simulink model "BFE_TestHarness"  (Simulink 8.6)
settings: Solver=FixedStepDiscrete  StartTime=0.0  StopTime=3  FixedStep=Ts  RelTol=1e-3
PreLoadFcn:
  | addpath('MBD_Tests')
  | 
  | load('Workspace\EnvVar.mat')
  | run('MBD_Tests\MBD_tests_init.m')
  | if exist('tl_preloadfcn','file'), tl_preloadfcn(gcs,402); end
PostLoadFcn:
  | if exist('tl_postloadfcn','file'), tl_postloadfcn(gcs,402); end
InitFcn:
  | if exist('tlds_init','file'), tlds_init(gcs); end
StartFcn:
  | if exist('tlds_start','file'), tlds_start(gcs); end
StopFcn:
  | if exist('tlds_stop','file'), tlds_stop(gcs); end
undefined symbols (not defined in the file): ddv, Ts, u2, u3, u4
libraries: tllib x11, simulink x8, LIB_TF_G_111 x2, LIB_TF_G_12_StepControl x2, LIB_TF_G_112 x1, LIB_TF_G_113 x1
(part 15 of 17)

== system BFE_TestHarness/BFE_AC_BeltFunctionExecution/Subsystem/BFE_AC_BeltFunctionExecution/BFE_AC_BeltFunctionExecution/BFE_runExecuteStandardSteps/ExecuteStandardSteps/SubsystemConvertOrderToMotorPower/Current_Regulation/Standard Regulation/RescaleMotorMeasure 1lsb = 50mA ==
  MotorCommandSign : Inport  RequirementInfo={} %GIDa_ddc2de95_3bef_4d8e_93b1_f33af8d229ea
  MotorUnsigned : Inport  RequirementInfo={} %GIDa_c6d26590_74e9_40ee_9fc6_c313c8b1f55d  Port=2
  0 Int 16bits : Constant  RequirementInfo={} %GIDa_7831c855_5c9d_4fc0_a40d_65f08d384ac0  Value=ddv('Common/KS16_ZERO')  OutDataTypeStr=uint8  mask(TL_Constant){data={'output',{'variable','Common/KS16_ZERO'},'date',735951.66853826388}}
      settings: CopyFcn=if exist('tl_reset_reviewflag','file')==2,tl_reset_reviewflag(gcbh);end  DeleteFcn=if exist('delete_tlblock','file')==2,delete_tlblock(gcbh);end  NameChangeFcn=if exist('rename_tlblock','file')==2,rename_tlblock(gcbh);end  OpenFcn=if exist('tl_open_blockdlg','file')==2,tl_open_blockdlg(gcbh);else,open_system(gcbh,'parameter');end
      mask Help: eval(['if exist(''tl_online_help'',''file'') == 2, tl_online_help(''Topic'',''TL_Constant''),else, web([''jar:file:///'',matlabroot,''/help/toolbox/simulink/help.jar!/slref/' lower(get_param(gcbh,'Blocktype')) '.html''], ''-helpbrowser''),end'])
      mask Display: plot([-0.05, 1.05, NaN, -0.05, 1.05],[.01, .01, NaN, .99, .99])
  BFE/KU8_PID_mA_RESCALING : Constant  RequirementInfo={} %GIDa_28865132_38f2_4152_8d2a_1d87ea42668e  Value=ddv('BFE/KU8_PID_mA_RESCALING')  OutDataTypeStr=uint8  mask(TL_Constant){data={'output',{'variable','BFE/KU8_PID_mA_RESCALING'},'date',735951.6685378704}}
      settings: CopyFcn=if exist('tl_reset_reviewflag','file')==2,tl_reset_reviewflag(gcbh);end  DeleteFcn=if exist('delete_tlblock','file')==2,delete_tlblock(gcbh);end  NameChangeFcn=if exist('rename_tlblock','file')==2,rename_tlblock(gcbh);end  OpenFcn=if exist('tl_open_blockdlg','file')==2,tl_open_blockdlg(gcbh);else,open_system(gcbh,'parameter');end
      mask Help: eval(['if exist(''tl_online_help'',''file'') == 2, tl_online_help(''Topic'',''TL_Constant''),else, web([''jar:file:///'',matlabroot,''/help/toolbox/simulink/help.jar!/slref/' lower(get_param(gcbh,'Blocktype')) '.html''], ''-helpbrowser''),end'])
      mask Display: plot([-0.05, 1.05, NaN, -0.05, 1.05],[.01, .01, NaN, .99, .99])
  KUC_ONE : Constant  RequirementInfo={} %GIDa_d9d69a7f_538e_4932_bf64_59549179e9a4  Value=ddv('Common/KU8_ONE')  OutDataTypeStr=uint8  mask(TL_Constant){data={'output',{'variable','Common/KU8_ONE'},'date',735951.66853748844}}
      settings: CopyFcn=if exist('tl_reset_reviewflag','file')==2,tl_reset_reviewflag(gcbh);end  DeleteFcn=if exist('delete_tlblock','file')==2,delete_tlblock(gcbh);end  NameChangeFcn=if exist('rename_tlblock','file')==2,rename_tlblock(gcbh);end  OpenFcn=if exist('tl_open_blockdlg','file')==2,tl_open_blockdlg(gcbh);else,open_system(gcbh,'parameter');end
      mask Help: eval(['if exist(''tl_online_help'',''file'') == 2, tl_online_help(''Topic'',''TL_Constant''),else, web([''jar:file:///'',matlabroot,''/help/toolbox/simulink/help.jar!/slref/' lower(get_param(gcbh,'Blocktype')) '.html''], ''-helpbrowser''),end'])
      mask Display: plot([-0.05, 1.05, NaN, -0.05, 1.05],[.01, .01, NaN, .99, .99])
  Product : Product  RequirementInfo={} %GIDa_989e5ae6_3fb7_483c_9c3c_230268316b82  Inputs=*/  OutDataTypeStr=uint32  RndMeth=Zero  mask(TL_Product){data={'output',{'type','UInt16'},'date',735951.66853710648}}
      settings: CopyFcn=if exist('tl_reset_reviewflag','file')==2,tl_reset_reviewflag(gcbh);end  DeleteFcn=if exist('delete_tlblock','file')==2,delete_tlblock(gcbh);end  NameChangeFcn=if exist('rename_tlblock','file')==2,rename_tlblock(gcbh);end  OpenFcn=if exist('tl_open_blockdlg','file')==2,tl_open_blockdlg(gcbh);else,open_system(gcbh,'parameter');end
      mask Help: eval(['if exist(''tl_online_help'',''file'') == 2, tl_online_help(''Topic'',''TL_Product''),else, web([''jar:file:///'',matlabroot,''/help/toolbox/simulink/help.jar!/slref/' lower(get_param(gcbh,'Blocktype')) '.html''], ''-helpbrowser''),end'])
      mask Display: plot([-0.05, 1.05, NaN, -0.05, 1.05],[.01, .01, NaN, .99, .99])
  Product1 : Product  RequirementInfo={} %GIDa_e457ca61_25f4_4aaf_857a_6a7a18ea8d4b  Inputs=**  OutDataTypeStr=int16  RndMeth=Zero  mask(TL_Product){data={'date',735951.66853673616}}
      settings: CopyFcn=if exist('tl_reset_reviewflag','file')==2,tl_reset_reviewflag(gcbh);end  DeleteFcn=if exist('delete_tlblock','file')==2,delete_tlblock(gcbh);end  NameChangeFcn=if exist('rename_tlblock','file')==2,rename_tlblock(gcbh);end  OpenFcn=if exist('tl_open_blockdlg','file')==2,tl_open_blockdlg(gcbh);else,open_system(gcbh,'parameter');end
      mask Help: eval(['if exist(''tl_online_help'',''file'') == 2, tl_online_help(''Topic'',''TL_Product''),else, web([''jar:file:///'',matlabroot,''/help/toolbox/simulink/help.jar!/slref/' lower(get_param(gcbh,'Blocktype')) '.html''], ''-helpbrowser''),end'])
      mask Display: plot([-0.05, 1.05, NaN, -0.05, 1.05],[.01, .01, NaN, .99, .99])
  Relational Operator : RelationalOperator  RequirementInfo={} %GIDa_0667d066_9ed8_4393_bb31_70e18b8dd437  Operator===  OutDataTypeStr=boolean  mask(TL_RelationalOperator){data={'date',735951.66853637737}}
      settings: DeleteFcn=if exist('delete_tlblock','file')==2,delete_tlblock(gcbh);end  NameChangeFcn=if exist('rename_tlblock','file')==2,rename_tlblock(gcbh);end  OpenFcn=if exist('tl_open_blockdlg','file')==2,tl_open_blockdlg(gcbh);else,open_system(gcbh,'parameter');end
      mask Help: eval(['if exist(''tl_online_help'',''file'') == 2, tl_online_help(''Topic'',''TL_RelationalOperator''),else, web([''jar:file:///'',matlabroot,''/help/toolbox/simulink/help.jar!/slref/' lower(get_param(gcbh,'Blocktype')) '.html''], ''-helpbrowser''),end'])
      mask Display: plot([-0.05, 1.05, NaN, -0.05, 1.05],[.01, .01, NaN, .99, .99])
  Sign : Signum  RequirementInfo={} %GIDa_e8c68066_07cd_49ad_8f47_c39297ac8a64  mask(TL_Signum){data={'date',735951.6685361343}}
      settings: DeleteFcn=if exist('delete_tlblock','file')==2,delete_tlblock(gcbh);end  NameChangeFcn=if exist('rename_tlblock','file')==2,rename_tlblock(gcbh);end  OpenFcn=if exist('tl_open_blockdlg','file')==2,tl_open_blockdlg(gcbh);else,open_system(gcbh,'parameter');end
      mask Help: eval(['if exist(''tl_online_help'',''file'') == 2, tl_online_help(''Topic'',''TL_Signum''),else, web([''jar:file:///'',matlabroot,''/help/toolbox/simulink/help.jar!/slref/' lower(get_param(gcbh,'Blocktype')) '.html''], ''-helpbrowser''),end'])
      mask Display: plot([-0.05, 1.05, NaN, -0.05, 1.05],[.01, .01, NaN, .99, .99])
  Switch : Switch  RequirementInfo={} %GIDa_e47adc39_9841_47d4_9acc_035cc38b4113  Criteria=u2 ~= 0  mask(TL_Switch){data={'output',{'type','Int8'},'date',735951.66853584489}}
      settings: CopyFcn=if exist('tl_reset_reviewflag','file')==2,tl_reset_reviewflag(gcbh);end  DeleteFcn=if exist('delete_tlblock','file')==2,delete_tlblock(gcbh);end  NameChangeFcn=if exist('rename_tlblock','file')==2,rename_tlblock(gcbh);end  OpenFcn=if exist('tl_open_blockdlg','file')==2,tl_open_blockdlg(gcbh);else,open_system(gcbh,'parameter');end
      mask Help: eval(['if exist(''tl_online_help'',''file'') == 2, tl_online_help(''Topic'',''TL_Switch''),else, web([''jar:file:///'',matlabroot,''/help/toolbox/simulink/help.jar!/slref/' lower(get_param(gcbh,'Blocktype')) '.html''], ''-helpbrowser''),end'])
      mask Display: plot([-0.05, 1.05, NaN, -0.05, 1.05],[.01, .01, NaN, .99, .99])
  s16MotorCurrent : Outport  RequirementInfo={} %GIDa_bea6628c_dfa8_47c5_b18b_49264848b5ef
  wires:
  MotorCommandSign/1 -> Sign/1, Relational Operator/2
  Sign/1 -> Switch/3
  0 Int 16bits/1 -> Relational Operator/1
  Relational Operator/1 -> Switch/2
  KUC_ONE/1 -> Switch/1
  Product/1 -> Product1/2
  Switch/1 -> Product1/1
  Product1/1 -> s16MotorCurrent/1
  MotorUnsigned/1 -> Product/1
  BFE/KU8_PID_mA_RESCALING/1 -> Product/2

== system BFE_TestHarness/BFE_AC_BeltFunctionExecution/Subsystem/BFE_AC_BeltFunctionExecution/BFE_AC_BeltFunctionExecution/BFE_runExecuteStandardSteps/ExecuteStandardSteps/SubsystemConvertOrderToMotorPower/RescaleOrderType/If Action Subsystem/8Bit Decoder ==
  U8in : Inport  RequirementInfo={} %GIDa_cca83995_da78_4ddb_b2c1_85f13c6d35e0
  8Bit Decoder : S-Function  RequirementInfo={} %GIDa_b6337983_b2e1_41bd_ae7f_dd9ba8b00acd  FunctionName=u8_bit_decoder_flp  Parameters=dt  SFunctionDeploymentMode=off  EnableBusSupport=off  mask(TL_CustomCode){data={'#state',0,'#param',0,'#work',0,'#output',8,'#logdata',8,'codefile','u8_bit_decoder.c','output#1',{'name','$S_$B_bit7','varname','bit7','type','Bool'},'output#2',{'name','$S_$B_bit6','varname','bit6','type','Bool'},'output#3',{'name','$S_$B_bit5','varname','bit5','type','Bool'},'output#4',{'name','$S_$B_bit4','varname','bit4','type','Bool'},'output#5',{'name','$S_$B_bit3','varname','bit3','type','Bool'},'output#6',{'name','$S_$B_bit2','varname','bit2','type','Bool'},'output#7',{'name','$S_$B_bit1','varname','bit1','type','Bool'},'output#8',{'name','$S_$B_bit0','varname','bit0','type','Bool'},'input',{'name','$S_$B_in','varname','u8in','type','UInt8'},'date',735951.66851649305}, dt=-1}
      mask help:
      | TargetLink Custom Code block:
      | Allows to insert custom code into a TargetLink application.
      settings: DeleteFcn=if exist('delete_tlblock','file')==2,delete_tlblock(gcbh);end  NameChangeFcn=if exist('rename_tlblock','file')==2,rename_tlblock(gcbh);end  OpenFcn=if exist('tl_open_blockdlg','file')==2,tl_open_blockdlg(gcbh);else,open_system(gcbh,'mask');end
      mask Help: eval('if exist(''tl_online_help'',''file'') == 2, tl_online_help(''Topic'',get_param(gcbh,''MaskType'')),end')
      mask Display:
      | plot([-0.05, 1.05, NaN, -0.05, 1.05],[.01, .01, NaN, .99, .99])
      | ; disp('u8_bit_decoder.c');port_label('input',1,'u8in');port_label('output',1,'bit7');port_label('output',2,'bit6');port_label('output',3,'bit5');port_label('output',4,'bit4');port_label('output',5,'bit3');port_label('output',6,'bit2');port_label('output',7,'bit1');port_label('output',8,'bit0');
  Bit7 : Outport  RequirementInfo={} %GIDa_79f6aec0_fcce_435d_ab59_8512532b1b11
  Bit6 : Outport  RequirementInfo={} %GIDa_7cd114c3_d211_44fb_b5cc_00bfdef86dbe  Port=2
  Bit5 : Outport  RequirementInfo={} %GIDa_012c8b96_621a_4aef_ba87_93ec05b55b0e  Port=3
  Bit4 : Outport  RequirementInfo={} %GIDa_16ec1885_4505_4833_8f08_779f3b6e4b74  Port=4
  Bit3 : Outport  RequirementInfo={} %GIDa_052869ce_db0b_4020_8a90_97f9c877a41f  Port=5
  Bit2 : Outport  RequirementInfo={} %GIDa_b38fc457_ade6_4ef7_baf3_aff089c2b6cc  Port=6
  Bit1 : Outport  RequirementInfo={} %GIDa_058fcc24_9702_4f94_b51b_68fafb1f5751  Port=7
  Bit0 : Outport  RequirementInfo={} %GIDa_08d7afe0_9577_46ee_bc11_f47871415acc  Port=8
  wires:
  8Bit Decoder/8 -> Bit0/1
  8Bit Decoder/7 -> Bit1/1
  8Bit Decoder/5 -> Bit3/1
  8Bit Decoder/4 -> Bit4/1
  8Bit Decoder/3 -> Bit5/1
  8Bit Decoder/2 -> Bit6/1
  8Bit Decoder/1 -> Bit7/1
  8Bit Decoder/6 -> Bit2/1
  U8in/1 -> 8Bit Decoder/1

== system BFE_TestHarness/BFE_AC_BeltFunctionExecution/Subsystem/BFE_AC_BeltFunctionExecution/BFE_AC_BeltFunctionExecution/BFE_runExecuteStandardSteps/ExecuteStandardSteps/SubsystemConvertOrderToMotorPower/RescaleOrderType/If Action Subsystem1/8Bit Decoder ==
  U8in : Inport  RequirementInfo={} %GIDa_f8d109da_a7cf_43cb_ba2a_57cff145f4b7
  8Bit Decoder : S-Function  RequirementInfo={} %GIDa_8480970b_d4f1_4300_8228_4b45f48dc331  FunctionName=u8_bit_decoder_flp  Parameters=dt  SFunctionDeploymentMode=off  EnableBusSupport=off  mask(TL_CustomCode){data={'#state',0,'#param',0,'#work',0,'#output',8,'#logdata',8,'codefile','u8_bit_decoder.c','output#1',{'name','$S_$B_bit7','varname','bit7','type','Bool'},'output#2',{'name','$S_$B_bit6','varname','bit6','type','Bool'},'output#3',{'name','$S_$B_bit5','varname','bit5','type','Bool'},'output#4',{'name','$S_$B_bit4','varname','bit4','type','Bool'},'output#5',{'name','$S_$B_bit3','varname','bit3','type','Bool'},'output#6',{'name','$S_$B_bit2','varname','bit2','type','Bool'},'output#7',{'name','$S_$B_bit1','varname','bit1','type','Bool'},'output#8',{'name','$S_$B_bit0','varname','bit0','type','Bool'},'input',{'name','$S_$B_in','varname','u8in','type','UInt8'},'date',735951.66851240746}, dt=-1}
      mask help:
      | TargetLink Custom Code block:
      | Allows to insert custom code into a TargetLink application.
      settings: DeleteFcn=if exist('delete_tlblock','file')==2,delete_tlblock(gcbh);end  NameChangeFcn=if exist('rename_tlblock','file')==2,rename_tlblock(gcbh);end  OpenFcn=if exist('tl_open_blockdlg','file')==2,tl_open_blockdlg(gcbh);else,open_system(gcbh,'mask');end
      mask Help: eval('if exist(''tl_online_help'',''file'') == 2, tl_online_help(''Topic'',get_param(gcbh,''MaskType'')),end')
      mask Display:
      | plot([-0.05, 1.05, NaN, -0.05, 1.05],[.01, .01, NaN, .99, .99])
      | ; disp('u8_bit_decoder.c');port_label('input',1,'u8in');port_label('output',1,'bit7');port_label('output',2,'bit6');port_label('output',3,'bit5');port_label('output',4,'bit4');port_label('output',5,'bit3');port_label('output',6,'bit2');port_label('output',7,'bit1');port_label('output',8,'bit0');
  Bit7 : Outport  RequirementInfo={} %GIDa_b6a5be25_b097_4284_bfb7_90bda14f7695
  Bit6 : Outport  RequirementInfo={} %GIDa_aa108eaf_6e73_4eff_ba0d_ce4b2cb6590f  Port=2
  Bit5 : Outport  RequirementInfo={} %GIDa_69d1ebf5_32de_4abe_9da7_6501e9c80693  Port=3
  Bit4 : Outport  RequirementInfo={} %GIDa_cff7f33f_15aa_4d45_9738_92334b2ad4cb  Port=4
  Bit3 : Outport  RequirementInfo={} %GIDa_10fb33c9_2c3b_4c51_9363_d2d49a1a57a5  Port=5
  Bit2 : Outport  RequirementInfo={} %GIDa_bbd0ff01_8027_4926_b455_dd681fe3b481  Port=6
  Bit1 : Outport  RequirementInfo={} %GIDa_bd4306cc_34c7_4243_b7f7_c39257ab2e00  Port=7
  Bit0 : Outport  RequirementInfo={} %GIDa_bf46a027_ea73_4fa1_ae0f_8a8120def989  Port=8
  wires:
  8Bit Decoder/8 -> Bit0/1
  8Bit Decoder/7 -> Bit1/1
  8Bit Decoder/5 -> Bit3/1
  8Bit Decoder/4 -> Bit4/1
  8Bit Decoder/3 -> Bit5/1
  8Bit Decoder/2 -> Bit6/1
  8Bit Decoder/1 -> Bit7/1
  8Bit Decoder/6 -> Bit2/1
  U8in/1 -> 8Bit Decoder/1

== system BFE_TestHarness/BFE_AC_BeltFunctionExecution/Subsystem/BFE_AC_BeltFunctionExecution/BFE_AC_BeltFunctionExecution/BFE_runExecuteStandardSteps/ExecuteStandardSteps/SubsystemConvertOrderToMotorPower/Current_Regulation/PID Regulation/PID feature enabled/DecidePID_Type ==
  bIsPIDSupplyAllowed : Inport  RequirementInfo={} %GIDa_b8e1bc41_3020_4f94_a10f_5d652f887f66
  bIsPIDMotorAllowed : Inport  RequirementInfo={} %GIDa_6b607d2d_643a_40f6_8b00_11a4c418d8d6  Port=2
  If : If  RequirementInfo={} %GIDa_f4e9c3ed_7e78_4540_80fe_45674d068906  NumInputs=2  IfExpression=u1  ElseIfExpressions=u2
  LastPIDType : Subsystem  RequirementInfo={} %GIDa_54517798_8ca0_4716_b2d4_af0f6596f023  TreatAsAtomicUnit=on
  Logical Operator : Logic  RequirementInfo={} %GIDa_3b220856_3c71_4e5e_b150_6d850348e8ad  AllPortsSameDT=off  OutDataTypeStr=boolean  mask(TL_LogicalOperator){data={'date',735951.66839079862}}
      settings: DeleteFcn=if exist('delete_tlblock','file')==2,delete_tlblock(gcbh);end  NameChangeFcn=if exist('rename_tlblock','file')==2,rename_tlblock(gcbh);end  OpenFcn=if exist('tl_open_blockdlg','file')==2,tl_open_blockdlg(gcbh);else,open_system(gcbh,'parameter');end
      mask Help: eval(['if exist(''tl_online_help'',''file'') == 2, tl_online_help(''Topic'',''TL_LogicalOperator''),else, web([''jar:file:///'',matlabroot,''/help/toolbox/simulink/help.jar!/slref/' lower(get_param(gcbh,'Blocktype')) '.html''], ''-helpbrowser''),end'])
      mask Display: plot([-0.05, 1.05, NaN, -0.05, 1.05],[.01, .01, NaN, .99, .99])
  Logical Operator1 : Logic  RequirementInfo={} %GIDa_73b78cc3_2296_4d3c_a902_7cc521734b54  Operator=NOT  Inputs=1  AllPortsSameDT=off  OutDataTypeStr=boolean  mask(TL_LogicalOperator){data={'date',735951.66839054401}}
      settings: DeleteFcn=if exist('delete_tlblock','file')==2,delete_tlblock(gcbh);end  NameChangeFcn=if exist('rename_tlblock','file')==2,rename_tlblock(gcbh);end  OpenFcn=if exist('tl_open_blockdlg','file')==2,tl_open_blockdlg(gcbh);else,open_system(gcbh,'parameter');end
      mask Help: eval(['if exist(''tl_online_help'',''file'') == 2, tl_online_help(''Topic'',''TL_LogicalOperator''),else, web([''jar:file:///'',matlabroot,''/help/toolbox/simulink/help.jar!/slref/' lower(get_param(gcbh,'Blocktype')) '.html''], ''-helpbrowser''),end'])
      mask Display: plot([-0.05, 1.05, NaN, -0.05, 1.05],[.01, .01, NaN, .99, .99])
  Logical Operator2 : Logic  RequirementInfo={} %GIDa_ca82c247_db8a_4876_a505_e83b3bf51f64  AllPortsSameDT=off  OutDataTypeStr=boolean  mask(TL_LogicalOperator){data={'date',735951.6683902893}}
      settings: DeleteFcn=if exist('delete_tlblock','file')==2,delete_tlblock(gcbh);end  NameChangeFcn=if exist('rename_tlblock','file')==2,rename_tlblock(gcbh);end  OpenFcn=if exist('tl_open_blockdlg','file')==2,tl_open_blockdlg(gcbh);else,open_system(gcbh,'parameter');end
      mask Help: eval(['if exist(''tl_online_help'',''file'') == 2, tl_online_help(''Topic'',''TL_LogicalOperator''),else, web([''jar:file:///'',matlabroot,''/help/toolbox/simulink/help.jar!/slref/' lower(get_param(gcbh,'Blocktype')) '.html''], ''-helpbrowser''),end'])
      mask Display: plot([-0.05, 1.05, NaN, -0.05, 1.05],[.01, .01, NaN, .99, .99])
  Logical Operator3 : Logic  RequirementInfo={} %GIDa_7a6df635_14d7_403c_9d76_c5868ae472fa  Operator=OR  AllPortsSameDT=off  OutDataTypeStr=boolean  mask(TL_LogicalOperator){data={'date',735951.6683900347}}
      settings: DeleteFcn=if exist('delete_tlblock','file')==2,delete_tlblock(gcbh);end  NameChangeFcn=if exist('rename_tlblock','file')==2,rename_tlblock(gcbh);end  OpenFcn=if exist('tl_open_blockdlg','file')==2,tl_open_blockdlg(gcbh);else,open_system(gcbh,'parameter');end
      mask Help: eval(['if exist(''tl_online_help'',''file'') == 2, tl_online_help(''Topic'',''TL_LogicalOperator''),else, web([''jar:file:///'',matlabroot,''/help/toolbox/simulink/help.jar!/slref/' lower(get_param(gcbh,'Blocktype')) '.html''], ''-helpbrowser''),end'])
      mask Display: plot([-0.05, 1.05, NaN, -0.05, 1.05],[.01, .01, NaN, .99, .99])
  Logical Operator4 : Logic  RequirementInfo={} %GIDa_61d74ce0_6e87_47a3_b109_464c73fdfd5c  AllPortsSameDT=off  OutDataTypeStr=boolean  mask(TL_LogicalOperator){data={'date',735951.66838979162}}
      settings: DeleteFcn=if exist('delete_tlblock','file')==2,delete_tlblock(gcbh);end  NameChangeFcn=if exist('rename_tlblock','file')==2,rename_tlblock(gcbh);end  OpenFcn=if exist('tl_open_blockdlg','file')==2,tl_open_blockdlg(gcbh);else,open_system(gcbh,'parameter');end
      mask Help: eval(['if exist(''tl_online_help'',''file'') == 2, tl_online_help(''Topic'',''TL_LogicalOperator''),else, web([''jar:file:///'',matlabroot,''/help/toolbox/simulink/help.jar!/slref/' lower(get_param(gcbh,'Blocktype')) '.html''], ''-helpbrowser''),end'])
      mask Display: plot([-0.05, 1.05, NaN, -0.05, 1.05],[.01, .01, NaN, .99, .99])
  Logical Operator5 : Logic  RequirementInfo={} %GIDa_40ce8f38_73a8_464c_90fe_5a3458c1d115  Operator=NOT  Inputs=1  AllPortsSameDT=off  OutDataTypeStr=boolean  mask(TL_LogicalOperator){data={'date',735951.66838953702}}
      settings: DeleteFcn=if exist('delete_tlblock','file')==2,delete_tlblock(gcbh);end  NameChangeFcn=if exist('rename_tlblock','file')==2,rename_tlblock(gcbh);end  OpenFcn=if exist('tl_open_blockdlg','file')==2,tl_open_blockdlg(gcbh);else,open_system(gcbh,'parameter');end
      mask Help: eval(['if exist(''tl_online_help'',''file'') == 2, tl_online_help(''Topic'',''TL_LogicalOperator''),else, web([''jar:file:///'',matlabroot,''/help/toolbox/simulink/help.jar!/slref/' lower(get_param(gcbh,'Blocktype')) '.html''], ''-helpbrowser''),end'])
      mask Display: plot([-0.05, 1.05, NaN, -0.05, 1.05],[.01, .01, NaN, .99, .99])
  Merge : Merge  RequirementInfo={} %GIDa_88d21688_780c_4457_9cb9_76f7f231122a  Inputs=3  InitialOutput=0  mask(TL_Merge){data={'output',{'name','u8PIDType','type','UInt8','inheritscaling',0},'date',735951.66838925926}}
      settings: CopyFcn=if exist('tl_reset_reviewflag','file')==2,tl_reset_reviewflag(gcbh);end  DeleteFcn=if exist('delete_tlblock','file')==2,delete_tlblock(gcbh);end  NameChangeFcn=if exist('rename_tlblock','file')==2,rename_tlblock(gcbh);end  OpenFcn=if exist('tl_open_blockdlg','file')==2,tl_open_blockdlg(gcbh);else,open_system(gcbh,'parameter');end
      mask Help: eval(['if exist(''tl_online_help'',''file'') == 2, tl_online_help(''Topic'',''TL_Merge''),else, web([''jar:file:///'',matlabroot,''/help/toolbox/simulink/help.jar!/slref/' lower(get_param(gcbh,'Blocktype')) '.html''], ''-helpbrowser''),end'])
      mask Display: plot([-0.05, 1.05, NaN, -0.05, 1.05],[.01, .01, NaN, .99, .99])
  MotorPID : Subsystem  RequirementInfo={} %GIDa_b0e18527_4ebe_420b_9ce9_04b6dc8075e8  TreatAsAtomicUnit=on
  SupplyPID : Subsystem  RequirementInfo={} %GIDa_5319e861_3821_4dd9_8e95_259230ced236  TreatAsAtomicUnit=on
  Unit Delay : UnitDelay  RequirementInfo={} %GIDa_20c92a67_2aef_4f74_a515_af7e0d9625f8  SampleTime=-1  mask(TL_UnitDelay){data={'output',{'type','UInt8'},'state',{'name','X_u8PreviousPIDtype','type','UInt8'},'date',735951.66838810185}}
      settings: CopyFcn=if exist('tl_reset_reviewflag','file')==2,tl_reset_reviewflag(gcbh);end  DeleteFcn=if exist('delete_tlblock','file')==2,delete_tlblock(gcbh);end  NameChangeFcn=if exist('rename_tlblock','file')==2,rename_tlblock(gcbh);end  OpenFcn=if exist('tl_open_blockdlg','file')==2,tl_open_blockdlg(gcbh);else,open_system(gcbh,'parameter');end
      mask Help: eval(['if exist(''tl_online_help'',''file'') == 2, tl_online_help(''Topic'',''TL_UnitDelay''),else, web([''jar:file:///'',matlabroot,''/help/toolbox/simulink/help.jar!/slref/' lower(get_param(gcbh,'Blocktype')) '.html''], ''-helpbrowser''),end'])
      mask Display: plot([-0.05, 1.05, NaN, -0.05, 1.05],[.01, .01, NaN, .99, .99])
  PID_Type : Outport  RequirementInfo={} %GIDa_a841a5ad_5add_402b_93f1_d11d6289a3f4
  wires:
  If/1 -> MotorPID/Action
  Merge/1 -> PID_Type/1, Unit Delay/1
  MotorPID/1(Out1) -> Merge/1
  SupplyPID/1(Out1) -> Merge/2
  LastPIDType/1(Out1) -> Merge/3
  If/2 -> SupplyPID/Action
  If/3 -> LastPIDType/Action
  Unit Delay/1 -> LastPIDType/1(In1)
  bIsPIDSupplyAllowed/1 -> Logical Operator1/1, Logical Operator2/2, Logical Operator4/2
  Logical Operator1/1 -> Logical Operator/2
  bIsPIDMotorAllowed/1 -> Logical Operator/1, Logical Operator5/1, Logical Operator4/1
  Logical Operator/1 -> If/1
  Logical Operator2/1 -> Logical Operator3/1
  Logical Operator4/1 -> Logical Operator3/2
  Logical Operator3/1 -> If/2
  Logical Operator5/1 -> Logical Operator2/1

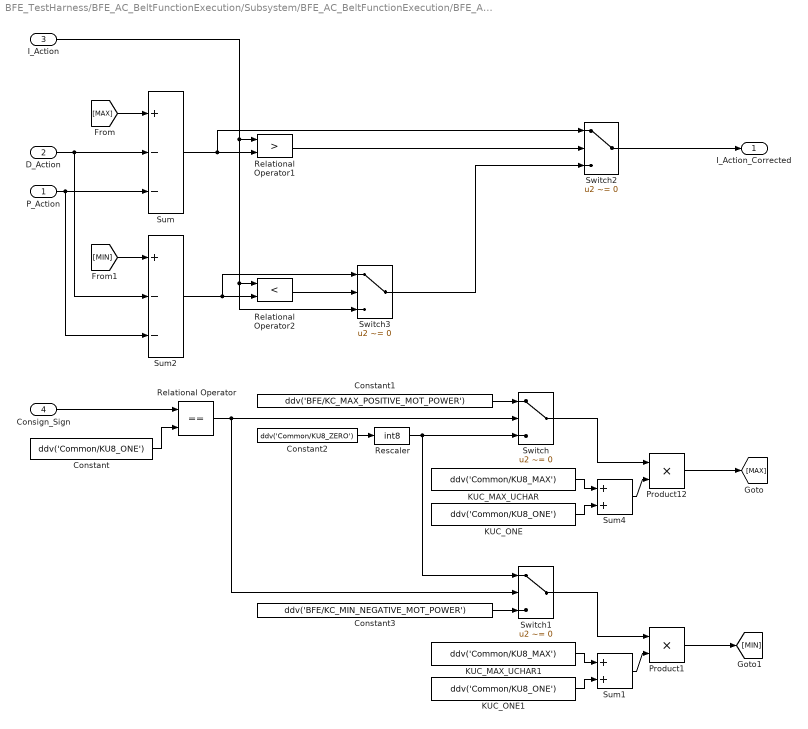
== system BFE_TestHarness/BFE_AC_BeltFunctionExecution/Subsystem/BFE_AC_BeltFunctionExecution/BFE_AC_BeltFunctionExecution/BFE_runExecuteStandardSteps/ExecuteStandardSteps/SubsystemConvertOrderToMotorPower/Current_Regulation/PID Regulation/PID feature enabled/Limit_Integer_Action ==
  P_Action : Inport  RequirementInfo={} %GIDa_07bf1ff6_2bcb_40d6_b65a_8be75430850f
  D_Action : Inport  RequirementInfo={} %GIDa_1a565a5c_b571_47d6_8429_7baedfea4a6f  Port=2
  I_Action : Inport  RequirementInfo={} %GIDa_6402cd07_c3b1_4ed5_a282_c846c1b94b00  Port=3
  Consign_Sign : Inport  RequirementInfo={} %GIDa_f88e813f_fe62_4969_bcbd_a80bfab87592  Port=4
  Constant : Constant  RequirementInfo={} %GIDa_3748518d_64b0_4891_a892_15491619f333  Value=ddv('Common/KU8_ONE')  OutDataTypeStr=uint8  mask(TL_Constant){data={'output',{'variable','Common/KU8_ONE'},'date',735951.6683844676}}
      settings: CopyFcn=if exist('tl_reset_reviewflag','file')==2,tl_reset_reviewflag(gcbh);end  DeleteFcn=if exist('delete_tlblock','file')==2,delete_tlblock(gcbh);end  NameChangeFcn=if exist('rename_tlblock','file')==2,rename_tlblock(gcbh);end  OpenFcn=if exist('tl_open_blockdlg','file')==2,tl_open_blockdlg(gcbh);else,open_system(gcbh,'parameter');end
      mask Help: eval(['if exist(''tl_online_help'',''file'') == 2, tl_online_help(''Topic'',''TL_Constant''),else, web([''jar:file:///'',matlabroot,''/help/toolbox/simulink/help.jar!/slref/' lower(get_param(gcbh,'Blocktype')) '.html''], ''-helpbrowser''),end'])
      mask Display: plot([-0.05, 1.05, NaN, -0.05, 1.05],[.01, .01, NaN, .99, .99])
  Constant1 : Constant  RequirementInfo={} %GIDa_9fcbdb90_a252_4ddd_af1d_ff9ca1d4857f  Value=ddv('BFE/KC_MAX_POSITIVE_MOT_POWER')  OutDataTypeStr=int8  mask(TL_Constant){data={'output',{'variable','BFE/KC_MAX_POSITIVE_MOT_POWER'},'date',735951.66838408564}}
      settings: CopyFcn=if exist('tl_reset_reviewflag','file')==2,tl_reset_reviewflag(gcbh);end  DeleteFcn=if exist('delete_tlblock','file')==2,delete_tlblock(gcbh);end  NameChangeFcn=if exist('rename_tlblock','file')==2,rename_tlblock(gcbh);end  OpenFcn=if exist('tl_open_blockdlg','file')==2,tl_open_blockdlg(gcbh);else,open_system(gcbh,'parameter');end
      mask Help: eval(['if exist(''tl_online_help'',''file'') == 2, tl_online_help(''Topic'',''TL_Constant''),else, web([''jar:file:///'',matlabroot,''/help/toolbox/simulink/help.jar!/slref/' lower(get_param(gcbh,'Blocktype')) '.html''], ''-helpbrowser''),end'])
      mask Display: plot([-0.05, 1.05, NaN, -0.05, 1.05],[.01, .01, NaN, .99, .99])
  Constant2 : Constant  RequirementInfo={} %GIDa_fa781778_632a_46ff_b4c3_26697425d789  Value=ddv('Common/KU8_ZERO')  OutDataTypeStr=int8  mask(TL_Constant){data={'output',{'variable','Common/KU8_ZERO'},'date',735951.66838373838}}
      settings: CopyFcn=if exist('tl_reset_reviewflag','file')==2,tl_reset_reviewflag(gcbh);end  DeleteFcn=if exist('delete_tlblock','file')==2,delete_tlblock(gcbh);end  NameChangeFcn=if exist('rename_tlblock','file')==2,rename_tlblock(gcbh);end  OpenFcn=if exist('tl_open_blockdlg','file')==2,tl_open_blockdlg(gcbh);else,open_system(gcbh,'parameter');end
      mask Help: eval(['if exist(''tl_online_help'',''file'') == 2, tl_online_help(''Topic'',''TL_Constant''),else, web([''jar:file:///'',matlabroot,''/help/toolbox/simulink/help.jar!/slref/' lower(get_param(gcbh,'Blocktype')) '.html''], ''-helpbrowser''),end'])
      mask Display: plot([-0.05, 1.05, NaN, -0.05, 1.05],[.01, .01, NaN, .99, .99])
  Constant3 : Constant  RequirementInfo={} %GIDa_73c79817_1942_43c8_ad20_ddf6c768f81d  Value=ddv('BFE/KC_MIN_NEGATIVE_MOT_POWER')  OutDataTypeStr=int8  mask(TL_Constant){data={'output',{'variable','BFE/KC_MIN_NEGATIVE_MOT_POWER'},'date',735951.66838336806}}
      settings: CopyFcn=if exist('tl_reset_reviewflag','file')==2,tl_reset_reviewflag(gcbh);end  DeleteFcn=if exist('delete_tlblock','file')==2,delete_tlblock(gcbh);end  NameChangeFcn=if exist('rename_tlblock','file')==2,rename_tlblock(gcbh);end  OpenFcn=if exist('tl_open_blockdlg','file')==2,tl_open_blockdlg(gcbh);else,open_system(gcbh,'parameter');end
      mask Help: eval(['if exist(''tl_online_help'',''file'') == 2, tl_online_help(''Topic'',''TL_Constant''),else, web([''jar:file:///'',matlabroot,''/help/toolbox/simulink/help.jar!/slref/' lower(get_param(gcbh,'Blocktype')) '.html''], ''-helpbrowser''),end'])
      mask Display: plot([-0.05, 1.05, NaN, -0.05, 1.05],[.01, .01, NaN, .99, .99])
  KUC_MAX_UCHAR : Constant  RequirementInfo={} %GIDa_9934e90a_7280_40c2_9e2e_e0ae95227e14  Value=ddv('Common/KU8_MAX')  OutDataTypeStr=uint8  mask(TL_Constant){data={'output',{'variable','Common/KU8_MAX'},'date',735951.66838300927}}
      settings: CopyFcn=if exist('tl_reset_reviewflag','file')==2,tl_reset_reviewflag(gcbh);end  DeleteFcn=if exist('delete_tlblock','file')==2,delete_tlblock(gcbh);end  NameChangeFcn=if exist('rename_tlblock','file')==2,rename_tlblock(gcbh);end  OpenFcn=if exist('tl_open_blockdlg','file')==2,tl_open_blockdlg(gcbh);else,open_system(gcbh,'parameter');end
      mask Help: eval(['if exist(''tl_online_help'',''file'') == 2, tl_online_help(''Topic'',''TL_Constant''),else, web([''jar:file:///'',matlabroot,''/help/toolbox/simulink/help.jar!/slref/' lower(get_param(gcbh,'Blocktype')) '.html''], ''-helpbrowser''),end'])
      mask Display: plot([-0.05, 1.05, NaN, -0.05, 1.05],[.01, .01, NaN, .99, .99])
  KUC_MAX_UCHAR1 : Constant  RequirementInfo={} %GIDa_1442abd7_3334_47c4_b88b_bf2df5825bef  Value=ddv('Common/KU8_MAX')  OutDataTypeStr=uint8  mask(TL_Constant){data={'output',{'variable','Common/KU8_MAX'},'date',735951.66838262731}}
      settings: CopyFcn=if exist('tl_reset_reviewflag','file')==2,tl_reset_reviewflag(gcbh);end  DeleteFcn=if exist('delete_tlblock','file')==2,delete_tlblock(gcbh);end  NameChangeFcn=if exist('rename_tlblock','file')==2,rename_tlblock(gcbh);end  OpenFcn=if exist('tl_open_blockdlg','file')==2,tl_open_blockdlg(gcbh);else,open_system(gcbh,'parameter');end
      mask Help: eval(['if exist(''tl_online_help'',''file'') == 2, tl_online_help(''Topic'',''TL_Constant''),else, web([''jar:file:///'',matlabroot,''/help/toolbox/simulink/help.jar!/slref/' lower(get_param(gcbh,'Blocktype')) '.html''], ''-helpbrowser''),end'])
      mask Display: plot([-0.05, 1.05, NaN, -0.05, 1.05],[.01, .01, NaN, .99, .99])
  KUC_ONE : Constant  RequirementInfo={} %GIDa_3798ea66_c8dd_4756_87ca_35ff58865d01  Value=ddv('Common/KU8_ONE')  OutDataTypeStr=uint8  mask(TL_Constant){data={'output',{'variable','Common/KU8_ONE'},'date',735951.66838225699}}
      settings: CopyFcn=if exist('tl_reset_reviewflag','file')==2,tl_reset_reviewflag(gcbh);end  DeleteFcn=if exist('delete_tlblock','file')==2,delete_tlblock(gcbh);end  NameChangeFcn=if exist('rename_tlblock','file')==2,rename_tlblock(gcbh);end  OpenFcn=if exist('tl_open_blockdlg','file')==2,tl_open_blockdlg(gcbh);else,open_system(gcbh,'parameter');end
      mask Help: eval(['if exist(''tl_online_help'',''file'') == 2, tl_online_help(''Topic'',''TL_Constant''),else, web([''jar:file:///'',matlabroot,''/help/toolbox/simulink/help.jar!/slref/' lower(get_param(gcbh,'Blocktype')) '.html''], ''-helpbrowser''),end'])
      mask Display: plot([-0.05, 1.05, NaN, -0.05, 1.05],[.01, .01, NaN, .99, .99])
  KUC_ONE1 : Constant  RequirementInfo={} %GIDa_93ab50c3_5730_4933_9310_989b40c14a9a  Value=ddv('Common/KU8_ONE')  OutDataTypeStr=uint8  mask(TL_Constant){data={'output',{'variable','Common/KU8_ONE'},'date',735951.66838186339}}
      settings: CopyFcn=if exist('tl_reset_reviewflag','file')==2,tl_reset_reviewflag(gcbh);end  DeleteFcn=if exist('delete_tlblock','file')==2,delete_tlblock(gcbh);end  NameChangeFcn=if exist('rename_tlblock','file')==2,rename_tlblock(gcbh);end  OpenFcn=if exist('tl_open_blockdlg','file')==2,tl_open_blockdlg(gcbh);else,open_system(gcbh,'parameter');end
      mask Help: eval(['if exist(''tl_online_help'',''file'') == 2, tl_online_help(''Topic'',''TL_Constant''),else, web([''jar:file:///'',matlabroot,''/help/toolbox/simulink/help.jar!/slref/' lower(get_param(gcbh,'Blocktype')) '.html''], ''-helpbrowser''),end'])
      mask Display: plot([-0.05, 1.05, NaN, -0.05, 1.05],[.01, .01, NaN, .99, .99])
  Product1 : Product  RequirementInfo={} %GIDa_a805d4aa_bf40_4c58_9fbb_1b9790d4bd60  Inputs=**  RndMeth=Zero  mask(TL_Product){data={'output',{'type','Int32'},'date',735951.66838146991}}
      settings: CopyFcn=if exist('tl_reset_reviewflag','file')==2,tl_reset_reviewflag(gcbh);end  DeleteFcn=if exist('delete_tlblock','file')==2,delete_tlblock(gcbh);end  NameChangeFcn=if exist('rename_tlblock','file')==2,rename_tlblock(gcbh);end  OpenFcn=if exist('tl_open_blockdlg','file')==2,tl_open_blockdlg(gcbh);else,open_system(gcbh,'parameter');end
      mask Help: eval(['if exist(''tl_online_help'',''file'') == 2, tl_online_help(''Topic'',''TL_Product''),else, web([''jar:file:///'',matlabroot,''/help/toolbox/simulink/help.jar!/slref/' lower(get_param(gcbh,'Blocktype')) '.html''], ''-helpbrowser''),end'])
      mask Display: plot([-0.05, 1.05, NaN, -0.05, 1.05],[.01, .01, NaN, .99, .99])
  Product12 : Product  RequirementInfo={} %GIDa_34672392_6764_48e2_8725_1abc846450b7  Inputs=**  RndMeth=Zero  mask(TL_Product){data={'output',{'type','Int32'},'date',735951.66838108795}}
      settings: CopyFcn=if exist('tl_reset_reviewflag','file')==2,tl_reset_reviewflag(gcbh);end  DeleteFcn=if exist('delete_tlblock','file')==2,delete_tlblock(gcbh);end  NameChangeFcn=if exist('rename_tlblock','file')==2,rename_tlblock(gcbh);end  OpenFcn=if exist('tl_open_blockdlg','file')==2,tl_open_blockdlg(gcbh);else,open_system(gcbh,'parameter');end
      mask Help: eval(['if exist(''tl_online_help'',''file'') == 2, tl_online_help(''Topic'',''TL_Product''),else, web([''jar:file:///'',matlabroot,''/help/toolbox/simulink/help.jar!/slref/' lower(get_param(gcbh,'Blocktype')) '.html''], ''-helpbrowser''),end'])
      mask Display: plot([-0.05, 1.05, NaN, -0.05, 1.05],[.01, .01, NaN, .99, .99])
  Relational Operator : RelationalOperator  RequirementInfo={} %GIDa_51c0bcc5_e4b7_4888_b2d3_efec1fb2f371  Operator===  OutDataTypeStr=boolean  mask(TL_RelationalOperator){data={'date',735951.66838072916}}
      settings: DeleteFcn=if exist('delete_tlblock','file')==2,delete_tlblock(gcbh);end  NameChangeFcn=if exist('rename_tlblock','file')==2,rename_tlblock(gcbh);end  OpenFcn=if exist('tl_open_blockdlg','file')==2,tl_open_blockdlg(gcbh);else,open_system(gcbh,'parameter');end
      mask Help: eval(['if exist(''tl_online_help'',''file'') == 2, tl_online_help(''Topic'',''TL_RelationalOperator''),else, web([''jar:file:///'',matlabroot,''/help/toolbox/simulink/help.jar!/slref/' lower(get_param(gcbh,'Blocktype')) '.html''], ''-helpbrowser''),end'])
      mask Display: plot([-0.05, 1.05, NaN, -0.05, 1.05],[.01, .01, NaN, .99, .99])
  Relational Operator1 : RelationalOperator  RequirementInfo={} %GIDa_6a535925_b9fb_40cb_bfbd_113cec544382  Operator=>  OutDataTypeStr=boolean  mask(TL_RelationalOperator){data={'date',735951.66838047456}}
      settings: DeleteFcn=if exist('delete_tlblock','file')==2,delete_tlblock(gcbh);end  NameChangeFcn=if exist('rename_tlblock','file')==2,rename_tlblock(gcbh);end  OpenFcn=if exist('tl_open_blockdlg','file')==2,tl_open_blockdlg(gcbh);else,open_system(gcbh,'parameter');end
      mask Help: eval(['if exist(''tl_online_help'',''file'') == 2, tl_online_help(''Topic'',''TL_RelationalOperator''),else, web([''jar:file:///'',matlabroot,''/help/toolbox/simulink/help.jar!/slref/' lower(get_param(gcbh,'Blocktype')) '.html''], ''-helpbrowser''),end'])
      mask Display: plot([-0.05, 1.05, NaN, -0.05, 1.05],[.01, .01, NaN, .99, .99])
  Relational Operator2 : RelationalOperator  RequirementInfo={} %GIDa_faa3725a_0264_47c3_9cb8_108a66a8fb09  Operator=<  OutDataTypeStr=boolean  mask(TL_RelationalOperator){data={'date',735951.66838023148}}
      settings: DeleteFcn=if exist('delete_tlblock','file')==2,delete_tlblock(gcbh);end  NameChangeFcn=if exist('rename_tlblock','file')==2,rename_tlblock(gcbh);end  OpenFcn=if exist('tl_open_blockdlg','file')==2,tl_open_blockdlg(gcbh);else,open_system(gcbh,'parameter');end
      mask Help: eval(['if exist(''tl_online_help'',''file'') == 2, tl_online_help(''Topic'',''TL_RelationalOperator''),else, web([''jar:file:///'',matlabroot,''/help/toolbox/simulink/help.jar!/slref/' lower(get_param(gcbh,'Blocktype')) '.html''], ''-helpbrowser''),end'])
      mask Display: plot([-0.05, 1.05, NaN, -0.05, 1.05],[.01, .01, NaN, .99, .99])
  Rescaler : DataTypeConversion  RequirementInfo={} %GIDa_d7c1b9fd_8334_479d_bf35_5b922f09031a  OutDataTypeStr=int8  SaturateOnIntegerOverflow=on  RndMeth=Zero  mask(TL_Rescaler){data={'output',{'type','Int8'},'date',735951.66837997688}}
      settings: DeleteFcn=if exist('delete_tlblock','file')==2,delete_tlblock(gcbh);end  NameChangeFcn=if exist('rename_tlblock','file')==2,rename_tlblock(gcbh);end  OpenFcn=if exist('tl_open_blockdlg','file')==2,tl_open_blockdlg(gcbh);else,open_system(gcbh,'parameter');end
      mask Help: eval(['if exist(''tl_online_help'',''file'') == 2, tl_online_help(''Topic'',''TL_Rescaler''),else, web([''jar:file:///'',matlabroot,''/help/toolbox/simulink/help.jar!/slref/' lower(get_param(gcbh,'Blocktype')) '.html''], ''-helpbrowser''),end'])
      mask Display: plot([-0.05, 1.05, NaN, -0.05, 1.05],[.01, .01, NaN, .99, .99])
  Sum : Sum  RequirementInfo={} %GIDa_81e2b2a7_7ff9_48cc_8413_04ade633cdbe  Inputs=+--  OutDataTypeStr=int32  mask(TL_Sum){data={'output',{'type','Int32'},'date',735951.66837965278}}
      settings: CopyFcn=if exist('tl_reset_reviewflag','file')==2,tl_reset_reviewflag(gcbh);end  DeleteFcn=if exist('delete_tlblock','file')==2,delete_tlblock(gcbh);end  NameChangeFcn=if exist('rename_tlblock','file')==2,rename_tlblock(gcbh);end  OpenFcn=if exist('tl_open_blockdlg','file')==2,tl_open_blockdlg(gcbh);else,open_system(gcbh,'parameter');end
      mask Help: eval(['if exist(''tl_online_help'',''file'') == 2, tl_online_help(''Topic'',''TL_Sum''),else, web([''jar:file:///'',matlabroot,''/help/toolbox/simulink/help.jar!/slref/' lower(get_param(gcbh,'Blocktype')) '.html''], ''-helpbrowser''),end'])
      mask Display: plot([-0.05, 1.05, NaN, -0.05, 1.05],[.01, .01, NaN, .99, .99])
  Sum1 : Sum  RequirementInfo={} %GIDa_3a01efc5_210f_4bab_9f2a_b95054b57c11  OutDataTypeStr=uint16  mask(TL_Sum){data={'output',{'type','UInt16'},'date',735951.66837929399}}
      settings: CopyFcn=if exist('tl_reset_reviewflag','file')==2,tl_reset_reviewflag(gcbh);end  DeleteFcn=if exist('delete_tlblock','file')==2,delete_tlblock(gcbh);end  NameChangeFcn=if exist('rename_tlblock','file')==2,rename_tlblock(gcbh);end  OpenFcn=if exist('tl_open_blockdlg','file')==2,tl_open_blockdlg(gcbh);else,open_system(gcbh,'parameter');end
      mask Help: eval(['if exist(''tl_online_help'',''file'') == 2, tl_online_help(''Topic'',''TL_Sum''),else, web([''jar:file:///'',matlabroot,''/help/toolbox/simulink/help.jar!/slref/' lower(get_param(gcbh,'Blocktype')) '.html''], ''-helpbrowser''),end'])
      mask Display: plot([-0.05, 1.05, NaN, -0.05, 1.05],[.01, .01, NaN, .99, .99])
  Sum2 : Sum  RequirementInfo={} %GIDa_ab9a0606_26e7_4408_a0ec_a71ed42a53b8  Inputs=+--  OutDataTypeStr=int32  mask(TL_Sum){data={'output',{'type','Int32'},'date',735951.6683789352}}
      settings: CopyFcn=if exist('tl_reset_reviewflag','file')==2,tl_reset_reviewflag(gcbh);end  DeleteFcn=if exist('delete_tlblock','file')==2,delete_tlblock(gcbh);end  NameChangeFcn=if exist('rename_tlblock','file')==2,rename_tlblock(gcbh);end  OpenFcn=if exist('tl_open_blockdlg','file')==2,tl_open_blockdlg(gcbh);else,open_system(gcbh,'parameter');end
      mask Help: eval(['if exist(''tl_online_help'',''file'') == 2, tl_online_help(''Topic'',''TL_Sum''),else, web([''jar:file:///'',matlabroot,''/help/toolbox/simulink/help.jar!/slref/' lower(get_param(gcbh,'Blocktype')) '.html''], ''-helpbrowser''),end'])
      mask Display: plot([-0.05, 1.05, NaN, -0.05, 1.05],[.01, .01, NaN, .99, .99])
  Sum4 : Sum  RequirementInfo={} %GIDa_26053b19_d989_4d2d_9417_ef435d71f101  OutDataTypeStr=uint16  mask(TL_Sum){data={'output',{'type','UInt16'},'date',735951.66837856476}}
      settings: CopyFcn=if exist('tl_reset_reviewflag','file')==2,tl_reset_reviewflag(gcbh);end  DeleteFcn=if exist('delete_tlblock','file')==2,delete_tlblock(gcbh);end  NameChangeFcn=if exist('rename_tlblock','file')==2,rename_tlblock(gcbh);end  OpenFcn=if exist('tl_open_blockdlg','file')==2,tl_open_blockdlg(gcbh);else,open_system(gcbh,'parameter');end
      mask Help: eval(['if exist(''tl_online_help'',''file'') == 2, tl_online_help(''Topic'',''TL_Sum''),else, web([''jar:file:///'',matlabroot,''/help/toolbox/simulink/help.jar!/slref/' lower(get_param(gcbh,'Blocktype')) '.html''], ''-helpbrowser''),end'])
      mask Display: plot([-0.05, 1.05, NaN, -0.05, 1.05],[.01, .01, NaN, .99, .99])
  Switch : Switch  RequirementInfo={} %GIDa_755939df_583a_4144_a379_00076e521599  Criteria=u2 ~= 0  mask(TL_Switch){data={'output',{'type','Int8'},'date',735951.66837817128}}
      settings: CopyFcn=if exist('tl_reset_reviewflag','file')==2,tl_reset_reviewflag(gcbh);end  DeleteFcn=if exist('delete_tlblock','file')==2,delete_tlblock(gcbh);end  NameChangeFcn=if exist('rename_tlblock','file')==2,rename_tlblock(gcbh);end  OpenFcn=if exist('tl_open_blockdlg','file')==2,tl_open_blockdlg(gcbh);else,open_system(gcbh,'parameter');end
      mask Help: eval(['if exist(''tl_online_help'',''file'') == 2, tl_online_help(''Topic'',''TL_Switch''),else, web([''jar:file:///'',matlabroot,''/help/toolbox/simulink/help.jar!/slref/' lower(get_param(gcbh,'Blocktype')) '.html''], ''-helpbrowser''),end'])
      mask Display: plot([-0.05, 1.05, NaN, -0.05, 1.05],[.01, .01, NaN, .99, .99])
  Switch1 : Switch  RequirementInfo={} %GIDa_8376b56b_3794_448d_ba47_aa33ee44ef44  Criteria=u2 ~= 0  mask(TL_Switch){data={'output',{'type','Int8'},'date',735951.66837765044}}
      settings: CopyFcn=if exist('tl_reset_reviewflag','file')==2,tl_reset_reviewflag(gcbh);end  DeleteFcn=if exist('delete_tlblock','file')==2,delete_tlblock(gcbh);end  NameChangeFcn=if exist('rename_tlblock','file')==2,rename_tlblock(gcbh);end  OpenFcn=if exist('tl_open_blockdlg','file')==2,tl_open_blockdlg(gcbh);else,open_system(gcbh,'parameter');end
      mask Help: eval(['if exist(''tl_online_help'',''file'') == 2, tl_online_help(''Topic'',''TL_Switch''),else, web([''jar:file:///'',matlabroot,''/help/toolbox/simulink/help.jar!/slref/' lower(get_param(gcbh,'Blocktype')) '.html''], ''-helpbrowser''),end'])
      mask Display: plot([-0.05, 1.05, NaN, -0.05, 1.05],[.01, .01, NaN, .99, .99])
  Switch2 : Switch  RequirementInfo={} %GIDa_b73be14d_0291_40ec_a371_db7764f57ee5  Criteria=u2 ~= 0  mask(TL_Switch){data={'output',{'type','Int32'},'date',735951.66837712959}}
      settings: CopyFcn=if exist('tl_reset_reviewflag','file')==2,tl_reset_reviewflag(gcbh);end  DeleteFcn=if exist('delete_tlblock','file')==2,delete_tlblock(gcbh);end  NameChangeFcn=if exist('rename_tlblock','file')==2,rename_tlblock(gcbh);end  OpenFcn=if exist('tl_open_blockdlg','file')==2,tl_open_blockdlg(gcbh);else,open_system(gcbh,'parameter');end
      mask Help: eval(['if exist(''tl_online_help'',''file'') == 2, tl_online_help(''Topic'',''TL_Switch''),else, web([''jar:file:///'',matlabroot,''/help/toolbox/simulink/help.jar!/slref/' lower(get_param(gcbh,'Blocktype')) '.html''], ''-helpbrowser''),end'])
      mask Display: plot([-0.05, 1.05, NaN, -0.05, 1.05],[.01, .01, NaN, .99, .99])
  Switch3 : Switch  RequirementInfo={} %GIDa_2753102e_4709_466f_80a7_db44eceb0853  Criteria=u2 ~= 0  mask(TL_Switch){data={'output',{'type','Int32'},'date',735951.66837659723}}
      settings: CopyFcn=if exist('tl_reset_reviewflag','file')==2,tl_reset_reviewflag(gcbh);end  DeleteFcn=if exist('delete_tlblock','file')==2,delete_tlblock(gcbh);end  NameChangeFcn=if exist('rename_tlblock','file')==2,rename_tlblock(gcbh);end  OpenFcn=if exist('tl_open_blockdlg','file')==2,tl_open_blockdlg(gcbh);else,open_system(gcbh,'parameter');end
      mask Help: eval(['if exist(''tl_online_help'',''file'') == 2, tl_online_help(''Topic'',''TL_Switch''),else, web([''jar:file:///'',matlabroot,''/help/toolbox/simulink/help.jar!/slref/' lower(get_param(gcbh,'Blocktype')) '.html''], ''-helpbrowser''),end'])
      mask Display: plot([-0.05, 1.05, NaN, -0.05, 1.05],[.01, .01, NaN, .99, .99])
  I_Action_Corrected : Outport  RequirementInfo={} %GIDa_482e1baf_681e_432e_a1ea_1cc7fccd2af7
  wires:
  Consign_Sign/1 -> Relational Operator/1
  Relational Operator/1 -> Switch/2, Switch1/2
  Constant/1 -> Relational Operator/2
  Constant1/1 -> Switch/1
  Constant2/1 -> Rescaler/1
  Constant3/1 -> Switch1/3
  KUC_MAX_UCHAR/1 -> Sum4/1
  KUC_ONE/1 -> Sum4/2
  Sum4/1 -> Product12/2
  Switch/1 -> Product12/1
  KUC_MAX_UCHAR1/1 -> Sum1/1
  KUC_ONE1/1 -> Sum1/2
  Sum1/1 -> Product1/2
  Switch1/1 -> Product1/1
  Product1/1 -> [MIN]
  Product12/1 -> [MAX]
  [MAX] -> Sum/1
  D_Action/1 -> Sum/2, Sum2/2
  P_Action/1 -> Sum/3, Sum2/3
  [MIN] -> Sum2/1
  Sum/1 -> Relational Operator1/2, Switch2/1
  I_Action/1 -> Relational Operator1/1, Relational Operator2/1, Switch3/3
  Sum2/1 -> Relational Operator2/2, Switch3/1
  Relational Operator1/1 -> Switch2/2
  Relational Operator2/1 -> Switch3/2
  Switch3/1 -> Switch2/3
  Switch2/1 -> I_Action_Corrected/1
  Rescaler/1 -> Switch/3, Switch1/1

== system BFE_TestHarness/BFE_AC_BeltFunctionExecution/Subsystem/BFE_AC_BeltFunctionExecution/BFE_AC_BeltFunctionExecution/BFE_runExecuteStandardSteps/ExecuteStandardSteps/SubsystemConvertOrderToMotorPower/Current_Regulation/PID Regulation/PID feature enabled/No_PID ==
  Action Port : ActionPort  RequirementInfo={} %GIDa_ef867887_64ae_4ad3_abfb_d91248d728d1  ActionType=default
  Gain : Gain  RequirementInfo={} %GIDa_9041e197_2ff8_458e_8836_b5da18c8b301  OutDataTypeStr=int32  mask(TL_Gain){data={'output',{'type','Int32'},'date',735951.66837190976}}
      settings: CopyFcn=if exist('tl_reset_reviewflag','file')==2,tl_reset_reviewflag(gcbh);end  DeleteFcn=if exist('delete_tlblock','file')==2,delete_tlblock(gcbh);end  NameChangeFcn=if exist('rename_tlblock','file')==2,rename_tlblock(gcbh);end  OpenFcn=if exist('tl_open_blockdlg','file')==2,tl_open_blockdlg(gcbh);else,open_system(gcbh,'parameter');end
      mask Help: eval(['if exist(''tl_online_help'',''file'') == 2, tl_online_help(''Topic'',''TL_Gain''),else, web([''jar:file:///'',matlabroot,''/help/toolbox/simulink/help.jar!/slref/' lower(get_param(gcbh,'Blocktype')) '.html''], ''-helpbrowser''),end'])
      mask Display: plot([0, .9, 0],[.05, .5, .95])
  Gain1 : Gain  RequirementInfo={} %GIDa_ddb249d0_b3cd_4084_b9e1_56cc76b8b0c6  OutDataTypeStr=int32  mask(TL_Gain){data={'output',{'type','Int32'},'date',735951.66837141209}}
      settings: CopyFcn=if exist('tl_reset_reviewflag','file')==2,tl_reset_reviewflag(gcbh);end  DeleteFcn=if exist('delete_tlblock','file')==2,delete_tlblock(gcbh);end  NameChangeFcn=if exist('rename_tlblock','file')==2,rename_tlblock(gcbh);end  OpenFcn=if exist('tl_open_blockdlg','file')==2,tl_open_blockdlg(gcbh);else,open_system(gcbh,'parameter');end
      mask Help: eval(['if exist(''tl_online_help'',''file'') == 2, tl_online_help(''Topic'',''TL_Gain''),else, web([''jar:file:///'',matlabroot,''/help/toolbox/simulink/help.jar!/slref/' lower(get_param(gcbh,'Blocktype')) '.html''], ''-helpbrowser''),end'])
      mask Display: plot([0, .9, 0],[.05, .5, .95])
  Gain2 : Gain  RequirementInfo={} %GIDa_edf65eb2_9ef0_4783_b4d0_6c38cd0df5cb  OutDataTypeStr=int32  mask(TL_Gain){data={'output',{'type','Int32'},'date',735951.6683709143}}
      settings: CopyFcn=if exist('tl_reset_reviewflag','file')==2,tl_reset_reviewflag(gcbh);end  DeleteFcn=if exist('delete_tlblock','file')==2,delete_tlblock(gcbh);end  NameChangeFcn=if exist('rename_tlblock','file')==2,rename_tlblock(gcbh);end  OpenFcn=if exist('tl_open_blockdlg','file')==2,tl_open_blockdlg(gcbh);else,open_system(gcbh,'parameter');end
      mask Help: eval(['if exist(''tl_online_help'',''file'') == 2, tl_online_help(''Topic'',''TL_Gain''),else, web([''jar:file:///'',matlabroot,''/help/toolbox/simulink/help.jar!/slref/' lower(get_param(gcbh,'Blocktype')) '.html''], ''-helpbrowser''),end'])
      mask Display: plot([0, .9, 0],[.05, .5, .95])
  KL_ZERO : Constant  RequirementInfo={} %GIDa_29eed0ba_cfc6_40bc_ba36_f364d977c63a  Value=ddv('Common/KS32_ZERO')  OutDataTypeStr=int32  mask(TL_Constant){data={'output',{'variable','Common/KS32_ZERO'},'date',735951.66837045143}}
      settings: CopyFcn=if exist('tl_reset_reviewflag','file')==2,tl_reset_reviewflag(gcbh);end  DeleteFcn=if exist('delete_tlblock','file')==2,delete_tlblock(gcbh);end  NameChangeFcn=if exist('rename_tlblock','file')==2,rename_tlblock(gcbh);end  OpenFcn=if exist('tl_open_blockdlg','file')==2,tl_open_blockdlg(gcbh);else,open_system(gcbh,'parameter');end
      mask Help: eval(['if exist(''tl_online_help'',''file'') == 2, tl_online_help(''Topic'',''TL_Constant''),else, web([''jar:file:///'',matlabroot,''/help/toolbox/simulink/help.jar!/slref/' lower(get_param(gcbh,'Blocktype')) '.html''], ''-helpbrowser''),end'])
      mask Display: plot([-0.05, 1.05, NaN, -0.05, 1.05],[.01, .01, NaN, .99, .99])
  s32P : Outport  RequirementInfo={} %GIDa_70513461_9af0_490e_8c56_77a68597a6a3  InitialOutput=0
  s32D : Outport  RequirementInfo={} %GIDa_d568bc7f_66b1_49f4_9ef7_9b91823c8c58  Port=2  InitialOutput=0
  s32I : Outport  RequirementInfo={} %GIDa_81f4627c_606b_49f2_bfee_7dcb91128927  Port=3  InitialOutput=0
  wires:
  KL_ZERO/1 -> Gain1/1, Gain2/1, Gain/1
  Gain/1 -> s32P/1
  Gain1/1 -> s32D/1
  Gain2/1 -> s32I/1
